simulink model "PassStCalib"  (R2024b)
settings: Solver=FixedStepDiscrete  StartTime=0.0  StopTime=10.0  FixedStep=0.01  RelTol=1e-3
model workspace (MAT data in the model file):
  KeSMSwAcsEntryPassStBkReclnUpwdDnwdPosMax_Val = Simulink.Parameter
  KeSMSwAcsEntryPassStBkReclnUpwdDnwdPosMax_Val.Value = 0
  KeSMSwAcsEntryPassStBkReclnUpwdDnwdPosMax_Val.Complexity = 'real'
  KeSMSwAcsEntryPassStBkReclnUpwdDnwdPosMax_Val.Dimensions = [1 1]
  KeSMSwAcsEntryPassStBkReclnUpwdDnwdPosMax_Val.DataType = 'uint16'
  KeSMSwAcsEntryPassStBkReclnUpwdDnwdPosMin_Val = Simulink.Parameter
  KeSMSwAcsEntryPassStBkReclnUpwdDnwdPosMin_Val.Value = 0
  KeSMSwAcsEntryPassStBkReclnUpwdDnwdPosMin_Val.Complexity = 'real'
  KeSMSwAcsEntryPassStBkReclnUpwdDnwdPosMin_Val.Dimensions = [1 1]
  KeSMSwAcsEntryPassStBkReclnUpwdDnwdPosMin_Val.DataType = 'uint16'
  KeSMSwAcsEntryPassStBkReclnUpwdDnwdPos_Val = Simulink.Parameter
  KeSMSwAcsEntryPassStBkReclnUpwdDnwdPos_Val.Value = 0
  KeSMSwAcsEntryPassStBkReclnUpwdDnwdPos_Val.Complexity = 'real'
  KeSMSwAcsEntryPassStBkReclnUpwdDnwdPos_Val.Dimensions = [1 1]
  KeSMSwAcsEntryPassStBkReclnUpwdDnwdPos_Val.DataType = 'uint16'
  KeSMSwAcsEntryPassStFrwdBkwdPosMax_Val = Simulink.Parameter
  KeSMSwAcsEntryPassStFrwdBkwdPosMax_Val.Value = 0
  KeSMSwAcsEntryPassStFrwdBkwdPosMax_Val.Complexity = 'real'
  KeSMSwAcsEntryPassStFrwdBkwdPosMax_Val.Dimensions = [1 1]
  KeSMSwAcsEntryPassStFrwdBkwdPosMax_Val.DataType = 'uint16'
  KeSMSwAcsEntryPassStFrwdBkwdPosMin_Val = Simulink.Parameter
  KeSMSwAcsEntryPassStFrwdBkwdPosMin_Val.Value = 0
  KeSMSwAcsEntryPassStFrwdBkwdPosMin_Val.Complexity = 'real'
  KeSMSwAcsEntryPassStFrwdBkwdPosMin_Val.Dimensions = [1 1]
  KeSMSwAcsEntryPassStFrwdBkwdPosMin_Val.DataType = 'uint16'
  KeSMSwAcsEntryPassStFrwdBkwdPos_Val = Simulink.Parameter
  KeSMSwAcsEntryPassStFrwdBkwdPos_Val.Value = 0
  KeSMSwAcsEntryPassStFrwdBkwdPos_Val.Complexity = 'real'
  KeSMSwAcsEntryPassStFrwdBkwdPos_Val.Dimensions = [1 1]
  KeSMSwAcsEntryPassStFrwdBkwdPos_Val.DataType = 'uint16'
  KeSMSwAcsMd56PassStBkReclnUpwdDnwdPosMax_Val = Simulink.Parameter
  KeSMSwAcsMd56PassStBkReclnUpwdDnwdPosMax_Val.Value = 0
  KeSMSwAcsMd56PassStBkReclnUpwdDnwdPosMax_Val.Complexity = 'real'
  KeSMSwAcsMd56PassStBkReclnUpwdDnwdPosMax_Val.Dimensions = [1 1]
  KeSMSwAcsMd56PassStBkReclnUpwdDnwdPosMax_Val.DataType = 'uint16'
  KeSMSwAcsMd56PassStBkReclnUpwdDnwdPosMin_Val = Simulink.Parameter
  KeSMSwAcsMd56PassStBkReclnUpwdDnwdPosMin_Val.Value = 0
  KeSMSwAcsMd56PassStBkReclnUpwdDnwdPosMin_Val.Complexity = 'real'
  KeSMSwAcsMd56PassStBkReclnUpwdDnwdPosMin_Val.Dimensions = [1 1]
  KeSMSwAcsMd56PassStBkReclnUpwdDnwdPosMin_Val.DataType = 'uint16'
  KeSMSwAcsMd56PassStBkReclnUpwdDnwdPos_Val = Simulink.Parameter
  KeSMSwAcsMd56PassStBkReclnUpwdDnwdPos_Val.Value = 0
  KeSMSwAcsMd56PassStBkReclnUpwdDnwdPos_Val.Complexity = 'real'
  KeSMSwAcsMd56PassStBkReclnUpwdDnwdPos_Val.Dimensions = [1 1]
  KeSMSwAcsMd56PassStBkReclnUpwdDnwdPos_Val.DataType = 'uint16'
  KeSMSwAcsMd56PassStFrwdBkwdPosMax_Val = Simulink.Parameter
  KeSMSwAcsMd56PassStFrwdBkwdPosMax_Val.Value = 0
  KeSMSwAcsMd56PassStFrwdBkwdPosMax_Val.Complexity = 'real'
  KeSMSwAcsMd56PassStFrwdBkwdPosMax_Val.Dimensions = [1 1]
  KeSMSwAcsMd56PassStFrwdBkwdPosMax_Val.DataType = 'uint16'
  KeSMSwAcsMd56PassStFrwdBkwdPosMin_Val = Simulink.Parameter
  KeSMSwAcsMd56PassStFrwdBkwdPosMin_Val.Value = 0
  KeSMSwAcsMd56PassStFrwdBkwdPosMin_Val.Complexity = 'real'
  KeSMSwAcsMd56PassStFrwdBkwdPosMin_Val.Dimensions = [1 1]
  KeSMSwAcsMd56PassStFrwdBkwdPosMin_Val.DataType = 'uint16'
  KeSMSwAcsMd56PassStFrwdBkwdPos_Val = Simulink.Parameter
  KeSMSwAcsMd56PassStFrwdBkwdPos_Val.Value = 0
  KeSMSwAcsMd56PassStFrwdBkwdPos_Val.Complexity = 'real'
  KeSMSwAcsMd56PassStFrwdBkwdPos_Val.Dimensions = [1 1]
  KeSMSwAcsMd56PassStFrwdBkwdPos_Val.DataType = 'uint16'
  KeSMSwRevRMDPassStBkReclnUpwdDnwdPosMax_Val = Simulink.Parameter
  KeSMSwRevRMDPassStBkReclnUpwdDnwdPosMax_Val.Value = 0
  KeSMSwRevRMDPassStBkReclnUpwdDnwdPosMax_Val.Complexity = 'real'
  KeSMSwRevRMDPassStBkReclnUpwdDnwdPosMax_Val.Dimensions = [1 1]
  KeSMSwRevRMDPassStBkReclnUpwdDnwdPosMax_Val.DataType = 'uint16'
  KeSMSwRevRMDPassStBkReclnUpwdDnwdPosMin_Val = Simulink.Parameter
  KeSMSwRevRMDPassStBkReclnUpwdDnwdPosMin_Val.Value = 0
  KeSMSwRevRMDPassStBkReclnUpwdDnwdPosMin_Val.Complexity = 'real'
  KeSMSwRevRMDPassStBkReclnUpwdDnwdPosMin_Val.Dimensions = [1 1]
  KeSMSwRevRMDPassStBkReclnUpwdDnwdPosMin_Val.DataType = 'uint16'
  KeSMSwRevRMDPassStBkReclnUpwdDnwdPos_Val = Simulink.Parameter
  KeSMSwRevRMDPassStBkReclnUpwdDnwdPos_Val.Value = 0
  KeSMSwRevRMDPassStBkReclnUpwdDnwdPos_Val.Complexity = 'real'
  KeSMSwRevRMDPassStBkReclnUpwdDnwdPos_Val.Dimensions = [1 1]
  KeSMSwRevRMDPassStBkReclnUpwdDnwdPos_Val.DataType = 'uint16'
  KeSMSwRevRMDPassStFrwdBkwdPosMax_Val = Simulink.Parameter
  KeSMSwRevRMDPassStFrwdBkwdPosMax_Val.Value = 0
  KeSMSwRevRMDPassStFrwdBkwdPosMax_Val.Complexity = 'real'
  KeSMSwRevRMDPassStFrwdBkwdPosMax_Val.Dimensions = [1 1]
  KeSMSwRevRMDPassStFrwdBkwdPosMax_Val.DataType = 'uint16'
  KeSMSwRevRMDPassStFrwdBkwdPosMin_Val = Simulink.Parameter
  KeSMSwRevRMDPassStFrwdBkwdPosMin_Val.Value = 0
  KeSMSwRevRMDPassStFrwdBkwdPosMin_Val.Complexity = 'real'
  KeSMSwRevRMDPassStFrwdBkwdPosMin_Val.Dimensions = [1 1]
  KeSMSwRevRMDPassStFrwdBkwdPosMin_Val.DataType = 'uint16'
  KeSMSwRevRMDPassStFrwdBkwdPos_Val = Simulink.Parameter
  KeSMSwRevRMDPassStFrwdBkwdPos_Val.Value = 0
  KeSMSwRevRMDPassStFrwdBkwdPos_Val.Complexity = 'real'
  KeSMSwRevRMDPassStFrwdBkwdPos_Val.Dimensions = [1 1]
  KeSMSwRevRMDPassStFrwdBkwdPos_Val.DataType = 'uint16'
undefined symbols (not defined in the file or in its folder): KeSMSuSecRwStVIPFtrstRefAngle_Val, KeSMSw6sAcsEntryPassStFtUpwdDnwdPos_Val, KeSMSw6sAcsEntryPassStFtUpwdDnwdPosMiax_Val, KeSMSw6sAcsEntryPassStFtUpwdDnwdPosMin_Val, KeSMSw6sAcsExtPassStFtUpwdDnwdPos_Val, KeSMSw6sAcsExtPassStFtUpwdDnwdPosMax_Val, KeSMSw6sAcsExtPassStFtUpwdDnwdPosMin_Val, KeSMSw6sRecoveryPassStStFtUpwdDnwdPos_Val, KeSMSw6sRecoveryPassStStFtUpwdDnwdPosMax_Val, KeSMSw6sRecoveryPassStStFtUpwdDnwdPosMin_Val, KeSMSw6SVIPMdPassStBkReclnUpwdDnwdPosPos_Val, KeSMSw6SVIPMdPassStBkReclnUpwdDnwdPosPosMax_Val, KeSMSw6SVIPMdPassStBkReclnUpwdDnwdPosPosMin_Val, KeSMSw6SVIPMdPassStFrwdBkwdPos2_Val, KeSMSw6SVIPMdPassStFrwdBkwdPosMax2_Val, KeSMSw6SVIPMdPassStFrwdBkwdPosMin2_Val, KeSMSw6SVIPMdPassStFrwdBkwdPosPos_Val, KeSMSw6SVIPMdPassStFrwdBkwdPosPosMax_Val, KeSMSw6SVIPMdPassStFrwdBkwdPosPosMin_Val, KeSMSwAcsEntryPassStFtUpwdDnwdPos_Val, KeSMSwAcsEntryPassStFtUpwdDnwdPosMiax_Val, KeSMSwAcsEntryPassStFtUpwdDnwdPosMin_Val, KeSMSwAcsExtPassStFtUpwdDnwdPos_Val, KeSMSwAcsExtPassStFtUpwdDnwdPosMax_Val, KeSMSwAcsExtPassStFtUpwdDnwdPosMin_Val, KeSMSwAcsMd30PassStBkReclnUpwdDnwdPos1_Val, KeSMSwAcsMd30PassStBkReclnUpwdDnwdPos1Max_Val, KeSMSwAcsMd30PassStBkReclnUpwdDnwdPos1Min_Val, KeSMSwAcsMd30PassStBkReclnUpwdDnwdPos_Val, KeSMSwAcsMd30PassStBkReclnUpwdDnwdPosMax_Val, KeSMSwAcsMd30PassStBkReclnUpwdDnwdPosMin_Val, KeSMSwAcsMd30PassStFldUpwdDnwdPos1_Val, KeSMSwAcsMd30PassStFldUpwdDnwdPos1Max_Val, KeSMSwAcsMd30PassStFldUpwdDnwdPos1Min_Val, KeSMSwAcsMd30PassStFldUpwdDnwdPos_Val, KeSMSwAcsMd30PassStFldUpwdDnwdPosMax_Val, KeSMSwAcsMd30PassStFldUpwdDnwdPosMin_Val, KeSMSwAcsMd30PassStFrwdBkwdPos1_Val, KeSMSwAcsMd30PassStFrwdBkwdPos1Max_Val, KeSMSwAcsMd30PassStFrwdBkwdPos1Min_Val, KeSMSwAcsMd30PassStFrwdBkwdPos_Val, KeSMSwAcsMd30PassStFrwdBkwdPosMax_Val, KeSMSwAcsMd30PassStFrwdBkwdPosMin_Val, KeSMSwAcsMd31PassStBkReclnUpwdDnwdPos1_Val, KeSMSwAcsMd31PassStBkReclnUpwdDnwdPos1Max_Val, KeSMSwAcsMd31PassStBkReclnUpwdDnwdPos1Min_Val, KeSMSwAcsMd31PassStBkReclnUpwdDnwdPos_Val, KeSMSwAcsMd31PassStBkReclnUpwdDnwdPosMax_Val, KeSMSwAcsMd31PassStBkReclnUpwdDnwdPosMin_Val, KeSMSwAcsMd31PassStFldUpwdDnwdPos_Val, KeSMSwAcsMd31PassStFldUpwdDnwdPosMax_Val, KeSMSwAcsMd31PassStFldUpwdDnwdPosMin_Val, KeSMSwAcsMd31PassStFrwdBkwdPos1_Val, KeSMSwAcsMd31PassStFrwdBkwdPos1Max_Val, KeSMSwAcsMd31PassStFrwdBkwdPos1Min_Val, KeSMSwAcsMd31PassStFrwdBkwdPos_Val, KeSMSwAcsMd31PassStFrwdBkwdPosMax_Val, KeSMSwAcsMd31PassStFrwdBkwdPosMin_Val, KeSMSwAcsMd57PassStBkReclnUpwdDnwdPosPos_Val, KeSMSwAcsMd57PassStBkReclnUpwdDnwdPosPosMax_Val ... (+34)
libraries: TrgtPosSelcLib x20
(part 1 of 3)
settings Model: ParameterArgumentNames=KeSMSwAcsEntryPassStBkReclnUpwdDnwdPosMax_Val,KeSMSwAcsEntryPassStBkReclnUpwdDnwdPosMin_Val,KeSMSwAcsEntryPassStBkReclnUpwdDnwdPos_Val,KeSMSwAcsEntryPassStFrwdBkwdPosMax_Val,KeSMSwAcsEntryPassStFrwdBkwdPosMin_Val,KeSMSwAcsEntryPassStFrwdBkwdPos_Val,KeSMSwAcsMd56PassStBkReclnUpwdDnwdPosMax_Val,KeSMSwAcsMd56PassStBkReclnUpwdDnwdPosMin_Val,KeSMSwAcsMd56PassStBkReclnUpwdDnwdPos_Val,KeSMSwAcsMd56PassStFrwdBkwdPosMax_Val,KeSMSwAcsMd56PassStFrwdBkwdPosMin_Val,KeSMSwAcsMd56PassStFrwdBkwdPos_Val,KeSMSwRevRMDPassStBkReclnUpwdDnwdPosMax_Val,KeSMSwRevRMDPassStBkReclnUpwdDnwdPosMin_Val,KeSMSwRevRMDPassStBkReclnUpwdDnwdPos_Val,KeSMSwRevRMDPassStFrwdBkwdPosMax_Val,KeSMSwRevRMDPassStFrwdBkwdPosMin_Val,KeSMSwRevRMDPassStFrwdBkwdPos_Val  Creator=sn2xws  LastModifiedBy=sn55gm
settings Model: ModifiedHistory=|
  | 2024.10.14 V3.0.0新增Md57，Md58
  | 2024.10.29 V3.0.1重新定义Unfold
  | 2024.11.6 V3.0.2 根据最新模式流程V2.6新增Md30 靠背位置1
  | 2024.11.18 V3.0.3 CR 946373 超级智享退出副驾改用Md31目标位置
  | 2024.11.27 V3.0.4 Md58 使用Md31的目标位置
  | 2024.12.11 V3.0.5 CR 953605
  | 2025.6.30 V3.13.0 新增Md61 md62
  | 25.7.31 V13.3.1 CR1100249 贵妃榻模式流程修改
settings SolverCC: AlgebraicLoopSolver=TrustRegion
settings DataIOCC: SaveFormat=StructureWithTime  ReturnWorkspaceOutputs=off
settings OptimizationCC: DefaultParameterBehavior=Inlined  EnhancedBackFolding=on  PassReuseOutputArgsAs=Individual arguments  ZeroExternalMemoryAtStartup=off  ZeroInternalMemoryAtStartup=off  OptimizeBlockOrder=speed  DifferentSizesBufferReuse=on  OptimizationCustomize=off  EfficientTunableParamExpr=on
settings DebuggingCC: ParameterTunabilityLossMsg=error  UnconnectedInputMsg=warning  UnconnectedOutputMsg=warning  UnconnectedLineMsg=warning  ArithmeticOperatorsInVariantConditions=warning
settings ModelReferenceCC: EnableRefExpFcnMdlSchedulingChecks=on
settings SFSimCC: MATLABDynamicMemAlloc=off  CustomCodeUndefinedFunction=UseInterfaceOnly
settings RTWCC: Description=AUTOSAR  SystemTargetFile=autosar.tlc  GenCodeOnly=on  TemplateMakefile=ert_default_tmf  GenerateReport=on  IncludeHyperlinkInReport=on  LaunchReport=on  DataTypeReplacement=CDataTypesFixedWidth  GenerateTraceInfo=on  GenerateTraceReport=on  GenerateTraceReportSl=on  GenerateTraceReportSf=on  GenerateTraceReportEml=on  GPUComputeCapability=3.5
settings CodeAppCC: ForceParamTrailComments=on  IgnoreCustomStorageClasses=off  OperatorAnnotations=on  SimulinkDataObjDesc=on  SFDataObjDesc=on  InsertBlockDesc=on
settings STFCustomTargetCC: TargetLangStandard=C99 (ISO)  MultiwordLength=256  ParMdlRefBuildCompliant=on  CompOptLevelCompliant=on  IncludeMdlTerminateFcn=off  CombineOutputUpdateFcns=on  SuppressErrorStatus=on  ERTCustomFileBanners=on  SupportNonFinite=off  SupportComplex=off  SupportContinuousTime=off  SupportNonInlinedSFcns=off  RemoveResetFunc=on  MATLABClassNameForMDSCustomization=Simulink.SoftwareTarget.ERTCustomization  AutosarCompliant=on  UseToolchainInfoCompliant=on  LookupTableObjectStructAxisOrder=2,1,3,4,...  LUTObjectStructOrderEvenSpacing=Size,Table,Breakpoints  SystemTargetFile=autosar.tlc
settings ERTTargetCC: TargetLangStandard=C99 (ISO)  ConcurrentExecutionCompliant=off  IncludeMdlTerminateFcn=off  SuppressErrorStatus=on  SupportNonFinite=off  SupportComplex=off  ModelStepFunctionPrototypeControlCompliant=off  CPPClassGenCompliant=off  AutosarCompliant=on  LookupTableObjectStructAxisOrder=2,1,3,4,...  LUTObjectStructOrderEvenSpacing=Size,Table,Breakpoints  ERTCustomFileTemplate=example_file_process.tlc  ERTFilePackagingFormat=Compact  BooleanTrueId=TRUE  BooleanFalseId=FALSE  DynamicArrayContainerType=coder::array

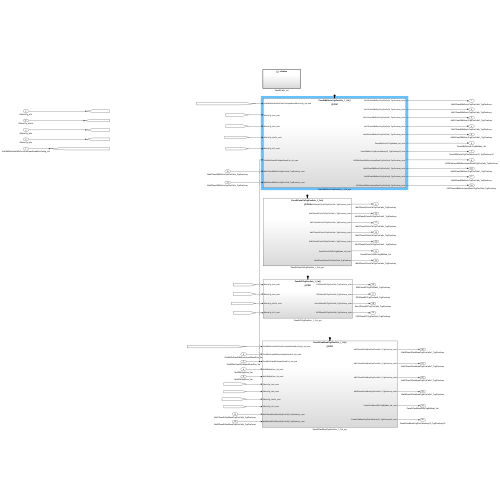
[thumbnail: Simulink's stored preview of the top-level diagram]
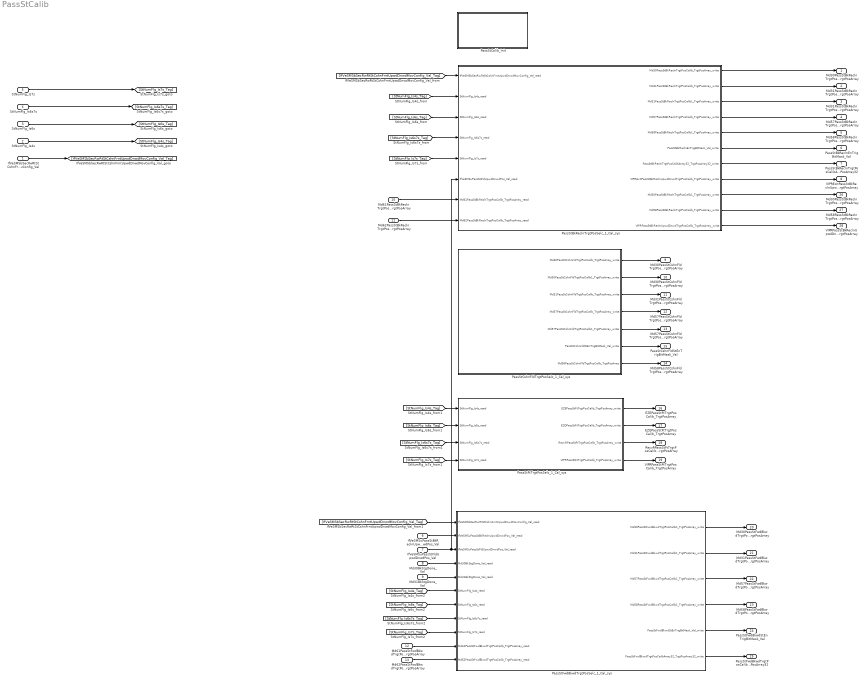
== system PassStCalib ==
  IfVeSMSbSecRwRtStCshnFrntUpwdDnwdMovConfig_Val : Inport  OutDataTypeStr=boolean  PortDimensions=1
  StNumFlg_Is4s : Inport  Port=2  OutDataTypeStr=boolean  PortDimensions=1
  StNumFlg_Is6s : Inport  Port=3  OutDataTypeStr=boolean  PortDimensions=1
  StNumFlg_Is6s7s : Inport  Port=4  OutDataTypeStr=boolean  PortDimensions=1
  StNumFlg_Is7s : Inport  Port=5  OutDataTypeStr=boolean  PortDimensions=1
  IfVeSMSuPassStBkReclnUpwdDnwdPos_Val : Inport  Port=6  OutDataTypeStr=uint16  PortDimensions=1
  IfVeSMSuPassStFldUpwdDnwdPos_Val : Inport  Port=7  OutDataTypeStr=uint16  PortDimensions=1
  Md30BkStgDone_Val : Inport  Port=8  OutDataTypeStr=boolean  PortDimensions=1
  Md31BkStgDone_Val : Inport  Port=9  OutDataTypeStr=boolean  PortDimensions=1
  Md61PassStBkReclnTrgtPosCalib_TrgtPosArray : Inport  Description=|  Port=10  OutDataTypeStr=uint16  PortDimensions=3
      | 0:Pos
      | 1:Max
      | 2:Min
  Md62PassStBkReclnTrgtPosCalib_TrgtPosArray : Inport  Description=|  Port=11  OutDataTypeStr=uint16  PortDimensions=3
      | 0:Pos
      | 1:Max
      | 2:Min
  Md61PassStFwdBkwdTrgtPosCalib_TrgtPosArray : Inport  Description=|  Port=12  OutDataTypeStr=uint16  PortDimensions=3
      | 0:Pos
      | 1:Max
      | 2:Min
  Md62PassStFwdBkwdTrgtPosCalib_TrgtPosArray : Inport  Description=|  Port=13  OutDataTypeStr=uint16  PortDimensions=3
      | 0:Pos
      | 1:Max
      | 2:Min
  PassStBkReclnTrgtPosSelc_1_Cal_sys : Subsystem
  PassStCalib_Init : Subsystem
  PassStCshnFldTrgtPosSelc_1_Cal_sys : Subsystem
  PassStFtTrgtPosSelc_1_Cal_sys : Subsystem
  PassStFwdBkwdTrgtPosSelc_1_Cal_sys : Subsystem
  Md30PassStBkReclnTrgtPosCalib_TrgtPosArray : Outport  Description=|  OutDataTypeStr=uint16  PortDimensions=3  VectorParamsAs1DForOutWhenUnconnected=off
      | 0:Pos
      | 1:Max
      | 2:Min
  Md31PassStBkReclnTrgtPosCalib_TrgtPosArray : Outport  Description=|  Port=2  OutDataTypeStr=uint16  PortDimensions=3  VectorParamsAs1DForOutWhenUnconnected=off
      | 0:Pos
      | 1:Max
      | 2:Min
  Md31PassStBkReclnTrgtPosCalib1_TrgtPosArray : Outport  Description=|  Port=3  OutDataTypeStr=uint16  PortDimensions=3  VectorParamsAs1DForOutWhenUnconnected=off
      | 0:Pos
      | 1:Max
      | 2:Min
  Md57PassStBkReclnTrgtPosCalib_TrgtPosArray : Outport  Description=|  Port=4  OutDataTypeStr=uint16  PortDimensions=3  VectorParamsAs1DForOutWhenUnconnected=off
      | 0:Pos
      | 1:Max
      | 2:Min
  Md58PassStBkReclnTrgtPosCalib1_TrgtPosArray : Outport  Description=|  Port=5  OutDataTypeStr=uint16  PortDimensions=3  VectorParamsAs1DForOutWhenUnconnected=off
      | 0:Pos
      | 1:Max
      | 2:Min
  PassStBkReclnEnTrigBitMask_Val : Outport  Port=6  OutDataTypeStr=uint32  PortDimensions=1  VectorParamsAs1DForOutWhenUnconnected=off
  PassStBkReclnTrgtPosCalibArray32_TrgtPosArray32 : Outport  Description=|  Port=7  OutDataTypeStr=uint16  PortDimensions=96  VectorParamsAs1DForOutWhenUnconnected=off
      | 0:Pos
      | 1:Max
      | 2:Min
  VIPRExitPassStBkReclnUpwdDnwdTrgtPosCalib_TrgtPosArray : Outport  Description=|  Port=8  OutDataTypeStr=uint16  PortDimensions=3  VectorParamsAs1DForOutWhenUnconnected=off
      | 0:Pos
      | 1:Max
      | 2:Min
  Md30PassStCshnFldTrgtPosCalib_TrgtPosArray : Outport  Description=|  Port=9  OutDataTypeStr=uint16  PortDimensions=3  VectorParamsAs1DForOutWhenUnconnected=off
      | 0:Pos
      | 1:Max
      | 2:Min
  Md30PassStCshnFldTrgtPosCalib1_TrgtPosArray : Outport  Description=|  Port=10  OutDataTypeStr=uint16  PortDimensions=3  VectorParamsAs1DForOutWhenUnconnected=off
      | 0:Pos
      | 1:Max
      | 2:Min
  Md31PassStCshnFldTrgtPosCalib_TrgtPosArray : Outport  Description=|  Port=11  OutDataTypeStr=uint16  PortDimensions=3  VectorParamsAs1DForOutWhenUnconnected=off
      | 0:Pos
      | 1:Max
      | 2:Min
  Md57PassStCshnFldTrgtPosCalib_TrgtPosArray : Outport  Description=|  Port=12  OutDataTypeStr=uint16  PortDimensions=3  VectorParamsAs1DForOutWhenUnconnected=off
      | 0:Pos
      | 1:Max
      | 2:Min
  Md57PassStCshnFldTrgtPosCalib1_TrgtPosArray : Outport  Description=|  Port=13  OutDataTypeStr=uint16  PortDimensions=3  VectorParamsAs1DForOutWhenUnconnected=off
      | 0:Pos
      | 1:Max
      | 2:Min
  Md58PassStCshnFldTrgtPosCalib_TrgtPosArray : Outport  Description=|  Port=14  OutDataTypeStr=uint16  PortDimensions=3  VectorParamsAs1DForOutWhenUnconnected=off
      | 0:Pos
      | 1:Max
      | 2:Min
  PassStCshnFldStEnTrigBitMask_Val : Outport  Port=15  OutDataTypeStr=uint32  PortDimensions=1  VectorParamsAs1DForOutWhenUnconnected=off
  EZEPassStFtTrgtPosCalib_TrgtPosArray : Outport  Description=|  Port=16  OutDataTypeStr=uint16  PortDimensions=3  VectorParamsAs1DForOutWhenUnconnected=off
      | 0:Pos
      | 1:Max
      | 2:Min
  EZQPassStFtTrgtPosCalib_TrgtPosArray : Outport  Description=|  Port=17  OutDataTypeStr=uint16  PortDimensions=3  VectorParamsAs1DForOutWhenUnconnected=off
      | 0:Pos
      | 1:Max
      | 2:Min
  RecvRPassStFtTrgtPosCalib_TrgtPosArray : Outport  Description=|  Port=18  OutDataTypeStr=uint16  PortDimensions=3  VectorParamsAs1DForOutWhenUnconnected=off
      | 0:Pos
      | 1:Max
      | 2:Min
  VIPRPassStFtTrgtPosCalib_TrgtPosArray : Outport  Description=|  Port=19  OutDataTypeStr=uint16  PortDimensions=3  VectorParamsAs1DForOutWhenUnconnected=off
      | 0:Pos
      | 1:Max
      | 2:Min
  Md30PassStFwdBkwdTrgtPosCalib1_TrgtPosArray : Outport  Description=|  Port=20  OutDataTypeStr=uint16  PortDimensions=3  VectorParamsAs1DForOutWhenUnconnected=off
      | 0:Pos
      | 1:Max
      | 2:Min
  Md31PassStFwdBkwdTrgtPosCalib1_TrgtPosArray : Outport  Description=|  Port=21  OutDataTypeStr=uint16  PortDimensions=3  VectorParamsAs1DForOutWhenUnconnected=off
      | 0:Pos
      | 1:Max
      | 2:Min
  Md57PassStFwdBkwdTrgtPosCalib1_TrgtPosArray : Outport  Description=|  Port=22  OutDataTypeStr=uint16  PortDimensions=3  VectorParamsAs1DForOutWhenUnconnected=off
      | 0:Pos
      | 1:Max
      | 2:Min
  Md58PassStFwdBkwdTrgtPosCalib1_TrgtPosArray : Outport  Description=|  Port=23  OutDataTypeStr=uint16  PortDimensions=3  VectorParamsAs1DForOutWhenUnconnected=off
      | 0:Pos
      | 1:Max
      | 2:Min
  PassStFwdBkwdStEnTrigBitMask_Val : Outport  Port=24  OutDataTypeStr=uint32  PortDimensions=1  VectorParamsAs1DForOutWhenUnconnected=off
  PassStFwdBkwdTrgtPosCalibArray32_TrgtPosArray32 : Outport  Description=|  Port=25  OutDataTypeStr=uint16  PortDimensions=96  VectorParamsAs1DForOutWhenUnconnected=off
      | 0:Pos
      | 1:Max
      | 2:Min
  Md30PassStBkReclnTrgtPosCalib1_TrgtPosArray : Outport  Description=|  Port=26  OutDataTypeStr=uint16  PortDimensions=3  VectorParamsAs1DForOutWhenUnconnected=off
      | 0:Pos
      | 1:Max
      | 2:Min
  Md58PassStBkReclnTrgtPosCalib_TrgtPosArray : Outport  Description=|  Port=27  OutDataTypeStr=uint16  PortDimensions=3  VectorParamsAs1DForOutWhenUnconnected=off
      | 0:Pos
      | 1:Max
      | 2:Min
  VIPRPassStBkReclnUpwdDnwdTrgtPosCalib_TrgtPosArray : Outport  Description=|  Port=28  OutDataTypeStr=uint16  PortDimensions=3  VectorParamsAs1DForOutWhenUnconnected=off
      | 0:Pos
      | 1:Max
      | 2:Min
  wires:
  PassStBkReclnTrgtPosSelc_1_Cal_sys/1(Md30PassStBkReclnTrgtPosCalib_TrgtPosArray_write) -> Md30PassStBkReclnTrgtPosCalib_TrgtPosArray/1
  PassStBkReclnTrgtPosSelc_1_Cal_sys/2(Md31PassStBkReclnTrgtPosCalib_TrgtPosArray_write) -> Md31PassStBkReclnTrgtPosCalib_TrgtPosArray/1
  PassStBkReclnTrgtPosSelc_1_Cal_sys/3(Md31PassStBkReclnTrgtPosCalib1_TrgtPosArray_write) -> Md31PassStBkReclnTrgtPosCalib1_TrgtPosArray/1
  PassStBkReclnTrgtPosSelc_1_Cal_sys/4(Md57PassStBkReclnTrgtPosCalib_TrgtPosArray_write) -> Md57PassStBkReclnTrgtPosCalib_TrgtPosArray/1
  PassStBkReclnTrgtPosSelc_1_Cal_sys/5(Md58PassStBkReclnTrgtPosCalib1_TrgtPosArray_write) -> Md58PassStBkReclnTrgtPosCalib1_TrgtPosArray/1
  PassStBkReclnTrgtPosSelc_1_Cal_sys/6(PassStBkReclnEnTrigBitMask_Val_write) -> PassStBkReclnEnTrigBitMask_Val/1
  PassStBkReclnTrgtPosSelc_1_Cal_sys/7(PassStBkReclnTrgtPosCalibArray32_TrgtPosArray32_write) -> PassStBkReclnTrgtPosCalibArray32_TrgtPosArray32/1
  PassStBkReclnTrgtPosSelc_1_Cal_sys/8(VIPRExitPassStBkReclnUpwdDnwdTrgtPosCalib_TrgtPosArray_write) -> VIPRExitPassStBkReclnUpwdDnwdTrgtPosCalib_TrgtPosArray/1
  PassStCshnFldTrgtPosSelc_1_Cal_sys/1(Md30PassStCshnFldTrgtPosCalib_TrgtPosArray_write) -> Md30PassStCshnFldTrgtPosCalib_TrgtPosArray/1
  PassStCshnFldTrgtPosSelc_1_Cal_sys/2(Md30PassStCshnFldTrgtPosCalib1_TrgtPosArray_write) -> Md30PassStCshnFldTrgtPosCalib1_TrgtPosArray/1
  PassStCshnFldTrgtPosSelc_1_Cal_sys/3(Md31PassStCshnFldTrgtPosCalib_TrgtPosArray_write) -> Md31PassStCshnFldTrgtPosCalib_TrgtPosArray/1
  PassStCshnFldTrgtPosSelc_1_Cal_sys/4(Md57PassStCshnFldTrgtPosCalib_TrgtPosArray_write) -> Md57PassStCshnFldTrgtPosCalib_TrgtPosArray/1
  PassStCshnFldTrgtPosSelc_1_Cal_sys/5(Md57PassStCshnFldTrgtPosCalib1_TrgtPosArray_write) -> Md57PassStCshnFldTrgtPosCalib1_TrgtPosArray/1
  PassStCshnFldTrgtPosSelc_1_Cal_sys/6(PassStCshnFldStEnTrigBitMask_Val_write) -> PassStCshnFldStEnTrigBitMask_Val/1
  PassStFtTrgtPosSelc_1_Cal_sys/1(EZEPassStFtTrgtPosCalib_TrgtPosArray_write) -> EZEPassStFtTrgtPosCalib_TrgtPosArray/1
  PassStFtTrgtPosSelc_1_Cal_sys/2(EZQPassStFtTrgtPosCalib_TrgtPosArray_write) -> EZQPassStFtTrgtPosCalib_TrgtPosArray/1
  PassStFtTrgtPosSelc_1_Cal_sys/3(RecvRPassStFtTrgtPosCalib_TrgtPosArray_write) -> RecvRPassStFtTrgtPosCalib_TrgtPosArray/1
  PassStFtTrgtPosSelc_1_Cal_sys/4(VIPRPassStFtTrgtPosCalib_TrgtPosArray_write) -> VIPRPassStFtTrgtPosCalib_TrgtPosArray/1
  IfVeSMSuPassStBkReclnUpwdDnwdPos_Val/1 -> PassStFwdBkwdTrgtPosSelc_1_Cal_sys/2(IfVeSMSuPassStBkReclnUpwdDnwdPos_Val_read)
  IfVeSMSuPassStFldUpwdDnwdPos_Val/1 -> PassStFwdBkwdTrgtPosSelc_1_Cal_sys/3(IfVeSMSuPassStFldUpwdDnwdPos_Val_read), PassStBkReclnTrgtPosSelc_1_Cal_sys/6(IfVeSMSuPassStFldUpwdDnwdPos_Val_read)
  Md30BkStgDone_Val/1 -> PassStFwdBkwdTrgtPosSelc_1_Cal_sys/4(Md30BkStgDone_Val_read)
  Md31BkStgDone_Val/1 -> PassStFwdBkwdTrgtPosSelc_1_Cal_sys/5(Md31BkStgDone_Val_read)
  PassStFwdBkwdTrgtPosSelc_1_Cal_sys/1(Md30PassStFwdBkwdTrgtPosCalib1_TrgtPosArray_write) -> Md30PassStFwdBkwdTrgtPosCalib1_TrgtPosArray/1
  PassStFwdBkwdTrgtPosSelc_1_Cal_sys/2(Md31PassStFwdBkwdTrgtPosCalib1_TrgtPosArray_write) -> Md31PassStFwdBkwdTrgtPosCalib1_TrgtPosArray/1
  PassStFwdBkwdTrgtPosSelc_1_Cal_sys/3(Md57PassStFwdBkwdTrgtPosCalib1_TrgtPosArray_write) -> Md57PassStFwdBkwdTrgtPosCalib1_TrgtPosArray/1
  PassStFwdBkwdTrgtPosSelc_1_Cal_sys/4(Md58PassStFwdBkwdTrgtPosCalib1_TrgtPosArray_write) -> Md58PassStFwdBkwdTrgtPosCalib1_TrgtPosArray/1
  PassStFwdBkwdTrgtPosSelc_1_Cal_sys/5(PassStFwdBkwdStEnTrigBitMask_Val_write) -> PassStFwdBkwdStEnTrigBitMask_Val/1
  PassStFwdBkwdTrgtPosSelc_1_Cal_sys/6(PassStFwdBkwdTrgtPosCalibArray32_TrgtPosArray32_write) -> PassStFwdBkwdTrgtPosCalibArray32_TrgtPosArray32/1
  StNumFlg_Is7s/1 -> [StNumFlg_Is7s_Tag]
  [StNumFlg_Is7s_Tag] -> PassStBkReclnTrgtPosSelc_1_Cal_sys/5(StNumFlg_Is7s_read)
  [StNumFlg_Is7s_Tag] -> PassStFtTrgtPosSelc_1_Cal_sys/4(StNumFlg_Is7s_read)
  [StNumFlg_Is7s_Tag] -> PassStFwdBkwdTrgtPosSelc_1_Cal_sys/9(StNumFlg_Is7s_read)
  StNumFlg_Is6s7s/1 -> [StNumFlg_Is6s7s_Tag]
  [StNumFlg_Is6s7s_Tag] -> PassStBkReclnTrgtPosSelc_1_Cal_sys/4(StNumFlg_Is6s7s_read)
  [StNumFlg_Is6s7s_Tag] -> PassStFtTrgtPosSelc_1_Cal_sys/3(StNumFlg_Is6s7s_read)
  [StNumFlg_Is6s7s_Tag] -> PassStFwdBkwdTrgtPosSelc_1_Cal_sys/8(StNumFlg_Is6s7s_read)
  StNumFlg_Is6s/1 -> [StNumFlg_Is6s_Tag]
  [StNumFlg_Is6s_Tag] -> PassStBkReclnTrgtPosSelc_1_Cal_sys/3(StNumFlg_Is6s_read)
  [StNumFlg_Is6s_Tag] -> PassStFtTrgtPosSelc_1_Cal_sys/2(StNumFlg_Is6s_read)
  [StNumFlg_Is6s_Tag] -> PassStFwdBkwdTrgtPosSelc_1_Cal_sys/7(StNumFlg_Is6s_read)
  StNumFlg_Is4s/1 -> [StNumFlg_Is4s_Tag]
  [StNumFlg_Is4s_Tag] -> PassStBkReclnTrgtPosSelc_1_Cal_sys/2(StNumFlg_Is4s_read)
  [StNumFlg_Is4s_Tag] -> PassStFtTrgtPosSelc_1_Cal_sys/1(StNumFlg_Is4s_read)
  [StNumFlg_Is4s_Tag] -> PassStFwdBkwdTrgtPosSelc_1_Cal_sys/6(StNumFlg_Is4s_read)
  IfVeSMSbSecRwRtStCshnFrntUpwdDnwdMovConfig_Val/1 -> [IfVeSMSbSecRwRtStCshnFrntUpwdDnwdMovConfig_Val_Tag]
  [IfVeSMSbSecRwRtStCshnFrntUpwdDnwdMovConfig_Val_Tag] -> PassStBkReclnTrgtPosSelc_1_Cal_sys/1(IfVeSMSbSecRwRtStCshnFrntUpwdDnwdMovConfig_Val_read)
  [IfVeSMSbSecRwRtStCshnFrntUpwdDnwdMovConfig_Val_Tag] -> PassStFwdBkwdTrgtPosSelc_1_Cal_sys/1(IfVeSMSbSecRwRtStCshnFrntUpwdDnwdMovConfig_Val_read)
  PassStBkReclnTrgtPosSelc_1_Cal_sys/9(Md30PassStBkReclnTrgtPosCalib1_TrgtPosArray_write) -> Md30PassStBkReclnTrgtPosCalib1_TrgtPosArray/1
  PassStBkReclnTrgtPosSelc_1_Cal_sys/10(Md58PassStBkReclnTrgtPosCalib_TrgtPosArray_write) -> Md58PassStBkReclnTrgtPosCalib_TrgtPosArray/1
  Md61PassStBkReclnTrgtPosCalib_TrgtPosArray/1 -> PassStBkReclnTrgtPosSelc_1_Cal_sys/7(Md61PassStBkReclnTrgtPosCalib_TrgtPosArray_read)
  Md62PassStBkReclnTrgtPosCalib_TrgtPosArray/1 -> PassStBkReclnTrgtPosSelc_1_Cal_sys/8(Md62PassStBkReclnTrgtPosCalib_TrgtPosArray_read)
  PassStBkReclnTrgtPosSelc_1_Cal_sys/11(VIPRPassStBkReclnUpwdDnwdTrgtPosCalib_TrgtPosArray_write) -> VIPRPassStBkReclnUpwdDnwdTrgtPosCalib_TrgtPosArray/1
  Md61PassStFwdBkwdTrgtPosCalib_TrgtPosArray/1 -> PassStFwdBkwdTrgtPosSelc_1_Cal_sys/10(Md61PassStFwdBkwdTrgtPosCalib_TrgtPosArray_read)
  Md62PassStFwdBkwdTrgtPosCalib_TrgtPosArray/1 -> PassStFwdBkwdTrgtPosSelc_1_Cal_sys/11(Md62PassStFwdBkwdTrgtPosCalib_TrgtPosArray_read)
  PassStCshnFldTrgtPosSelc_1_Cal_sys/7(Md58PassStCshnFldTrgtPosCalib_TrgtPosArray) -> Md58PassStCshnFldTrgtPosCalib_TrgtPosArray/1

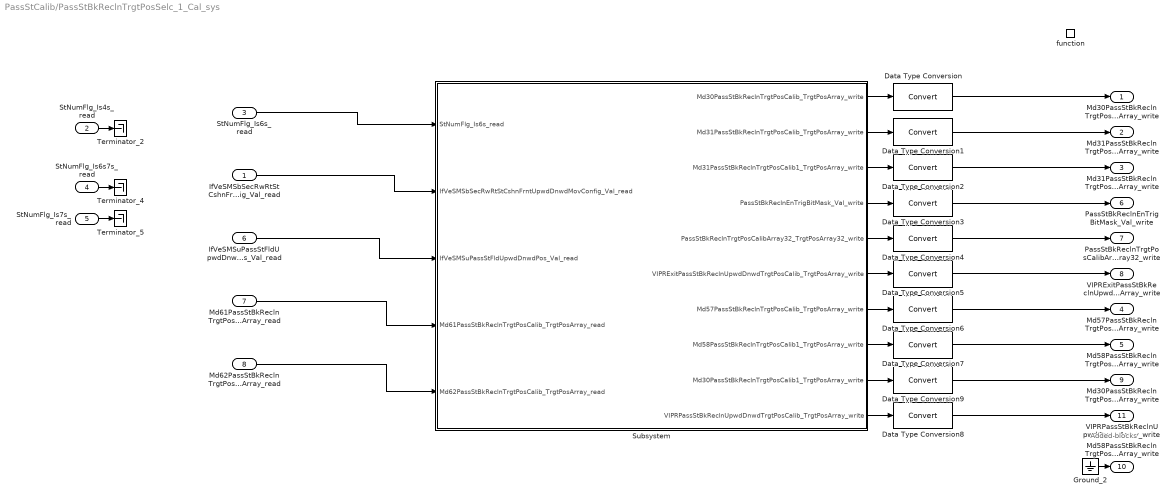
== system PassStCalib/PassStBkReclnTrgtPosSelc_1_Cal_sys ==
  note: Added blocks
  IfVeSMSbSecRwRtStCshnFrntUpwdDnwdMovConfig_Val_read : Inport
  StNumFlg_Is4s_read : Inport  Port=2
  StNumFlg_Is6s_read : Inport  Port=3
  StNumFlg_Is6s7s_read : Inport  Port=4
  StNumFlg_Is7s_read : Inport  Port=5
  IfVeSMSuPassStFldUpwdDnwdPos_Val_read : Inport  Port=6
  Md61PassStBkReclnTrgtPosCalib_TrgtPosArray_read : Inport  Port=7
  Md62PassStBkReclnTrgtPosCalib_TrgtPosArray_read : Inport  Port=8
  function : TriggerPort  TriggerType=function-call  IsSimulinkFunction=on  FunctionName=PassStBkReclnTrgtPosSelc_1_Cal  VariantControl=(inherit)
  Data Type Conversion{,1..9} (10 alike) : DataTypeConversion  SaturateOnIntegerOverflow=off  RndMeth=Floor
  Ground_2 : Ground
  Subsystem : Subsystem
  Terminator_2 : Terminator
  Terminator_4 : Terminator
  Terminator_5 : Terminator
  Md30PassStBkReclnTrgtPosCalib_TrgtPosArray_write : Outport  VectorParamsAs1DForOutWhenUnconnected=off
  Md31PassStBkReclnTrgtPosCalib_TrgtPosArray_write : Outport  Port=2  VectorParamsAs1DForOutWhenUnconnected=off
  Md31PassStBkReclnTrgtPosCalib1_TrgtPosArray_write : Outport  Port=3  VectorParamsAs1DForOutWhenUnconnected=off
  Md57PassStBkReclnTrgtPosCalib_TrgtPosArray_write : Outport  Port=4  VectorParamsAs1DForOutWhenUnconnected=off
  Md58PassStBkReclnTrgtPosCalib1_TrgtPosArray_write : Outport  Port=5  VectorParamsAs1DForOutWhenUnconnected=off
  PassStBkReclnEnTrigBitMask_Val_write : Outport  Port=6  VectorParamsAs1DForOutWhenUnconnected=off
  PassStBkReclnTrgtPosCalibArray32_TrgtPosArray32_write : Outport  Port=7  VectorParamsAs1DForOutWhenUnconnected=off
  VIPRExitPassStBkReclnUpwdDnwdTrgtPosCalib_TrgtPosArray_write : Outport  Port=8  VectorParamsAs1DForOutWhenUnconnected=off
  Md30PassStBkReclnTrgtPosCalib1_TrgtPosArray_write : Outport  Port=9  VectorParamsAs1DForOutWhenUnconnected=off
  Md58PassStBkReclnTrgtPosCalib_TrgtPosArray_write : Outport  Port=10  VectorParamsAs1DForOutWhenUnconnected=off
  VIPRPassStBkReclnUpwdDnwdTrgtPosCalib_TrgtPosArray_write : Outport  Port=11  VectorParamsAs1DForOutWhenUnconnected=off
      settings: EnsureOutportIsVirtual=on
  wires:
  IfVeSMSbSecRwRtStCshnFrntUpwdDnwdMovConfig_Val_read/1 -> Subsystem/2(IfVeSMSbSecRwRtStCshnFrntUpwdDnwdMovConfig_Val_read)
  StNumFlg_Is4s_read/1 -> Terminator_2/1
  StNumFlg_Is6s_read/1 -> Subsystem/1(StNumFlg_Is6s_read)
  StNumFlg_Is6s7s_read/1 -> Terminator_4/1
  StNumFlg_Is7s_read/1 -> Terminator_5/1
  Subsystem/1(Md30PassStBkReclnTrgtPosCalib_TrgtPosArray_write) -> Data Type Conversion/1
  Subsystem/2(Md31PassStBkReclnTrgtPosCalib_TrgtPosArray_write) -> Data Type Conversion1/1
  Subsystem/3(Md31PassStBkReclnTrgtPosCalib1_TrgtPosArray_write) -> Data Type Conversion2/1
  Subsystem/4(PassStBkReclnEnTrigBitMask_Val_write) -> Data Type Conversion3/1
  Subsystem/5(PassStBkReclnTrgtPosCalibArray32_TrgtPosArray32_write) -> Data Type Conversion4/1
  Subsystem/6(VIPRExitPassStBkReclnUpwdDnwdTrgtPosCalib_TrgtPosArray_write) -> Data Type Conversion5/1
  Subsystem/7(Md57PassStBkReclnTrgtPosCalib_TrgtPosArray_write) -> Data Type Conversion6/1
  Subsystem/8(Md58PassStBkReclnTrgtPosCalib1_TrgtPosArray_write) -> Data Type Conversion7/1
  Data Type Conversion/1 -> Md30PassStBkReclnTrgtPosCalib_TrgtPosArray_write/1
  Data Type Conversion1/1 -> Md31PassStBkReclnTrgtPosCalib_TrgtPosArray_write/1
  Data Type Conversion2/1 -> Md31PassStBkReclnTrgtPosCalib1_TrgtPosArray_write/1
  Data Type Conversion3/1 -> PassStBkReclnEnTrigBitMask_Val_write/1
  Data Type Conversion4/1 -> PassStBkReclnTrgtPosCalibArray32_TrgtPosArray32_write/1
  Data Type Conversion5/1 -> VIPRExitPassStBkReclnUpwdDnwdTrgtPosCalib_TrgtPosArray_write/1
  Data Type Conversion6/1 -> Md57PassStBkReclnTrgtPosCalib_TrgtPosArray_write/1
  Data Type Conversion7/1 -> Md58PassStBkReclnTrgtPosCalib1_TrgtPosArray_write/1
  Subsystem/9(Md30PassStBkReclnTrgtPosCalib1_TrgtPosArray_write) -> Data Type Conversion9/1
  Ground_2/1 -> Md58PassStBkReclnTrgtPosCalib_TrgtPosArray_write/1
  IfVeSMSuPassStFldUpwdDnwdPos_Val_read/1 -> Subsystem/3(IfVeSMSuPassStFldUpwdDnwdPos_Val_read)
  Data Type Conversion9/1 -> Md30PassStBkReclnTrgtPosCalib1_TrgtPosArray_write/1
  Md61PassStBkReclnTrgtPosCalib_TrgtPosArray_read/1 -> Subsystem/4(Md61PassStBkReclnTrgtPosCalib_TrgtPosArray_read)
  Md62PassStBkReclnTrgtPosCalib_TrgtPosArray_read/1 -> Subsystem/5(Md62PassStBkReclnTrgtPosCalib_TrgtPosArray_read)
  Subsystem/10(VIPRPassStBkReclnUpwdDnwdTrgtPosCalib_TrgtPosArray_write) -> Data Type Conversion8/1
  Data Type Conversion8/1 -> VIPRPassStBkReclnUpwdDnwdTrgtPosCalib_TrgtPosArray_write/1

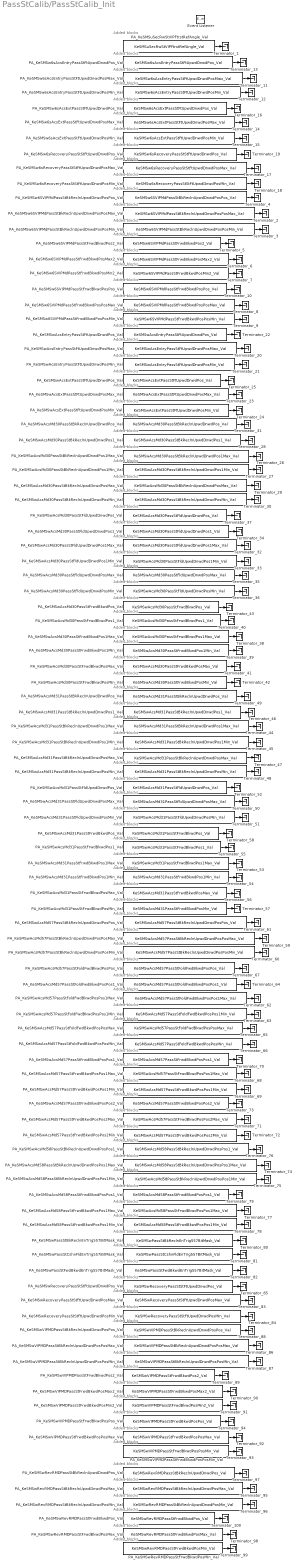
== system PassStCalib/PassStCalib_Init ==
  note: Added blocks
  note: Added blocks
  note: Added blocks
  note: Added blocks
  note: Added blocks
  note: Added blocks
  note: Added blocks
  note: Added blocks
  note: Added blocks
  note: Added blocks
  note: Added blocks
  note: Added blocks
  note: Added blocks
  note: Added blocks
  note: Added blocks
  note: Added blocks
  note: Added blocks
  note: Added blocks
  note: Added blocks
  note: Added blocks
  note: Added blocks
  note: Added blocks
  note: Added blocks
  note: Added blocks
  note: Added blocks
  note: Added blocks
  note: Added blocks
  note: Added blocks
  note: Added blocks
  note: Added blocks
  note: Added blocks
  note: Added blocks
  note: Added blocks
  note: Added blocks
  note: Added blocks
  note: Added blocks
  note: Added blocks
  note: Added blocks
  note: Added blocks
  note: Added blocks
  note: Added blocks
  note: Added blocks
  note: Added blocks
  note: Added blocks
  note: Added blocks
  note: Added blocks
  note: Added blocks
  note: Added blocks
  note: Added blocks
  note: Added blocks
  note: Added blocks
  note: Added blocks
  note: Added blocks
  note: Added blocks
  note: Added blocks
  note: Added blocks
  note: Added blocks
  note: Added blocks
  note: Added blocks
  note: Added blocks
  note: Added blocks
  note: Added blocks
  note: Added blocks
  note: Added blocks
  note: Added blocks
  note: Added blocks
  note: Added blocks
  note: Added blocks
  note: Added blocks
  note: Added blocks
  note: Added blocks
  note: Added blocks
  note: Added blocks
  note: Added blocks
  note: Added blocks
  note: Added blocks
  note: Added blocks
  note: Added blocks
  note: Added blocks
  note: Added blocks
  note: Added blocks
  note: Added blocks
  note: Added blocks
  note: Added blocks
  note: Added blocks
  note: Added blocks
  note: Added blocks
  note: Added blocks
  note: Added blocks
  note: Added blocks
  note: Added blocks
  note: Added blocks
  note: Added blocks
  note: Added blocks
  note: Added blocks
  note: Added blocks
  note: Added blocks
  note: Added blocks
  note: Added blocks
  note: Added blocks
  Event Listener : EventListener  EventName=reset
  PA_KeSMSuSecRwStVIPFtrstRefAngle_Val : Constant  Value=KeSMSuSecRwStVIPFtrstRefAngle_Val
  PA_KeSMSw6SVIPMdPassStBkReclnUpwdDnwdPosPosMax_Val : Constant  Value=KeSMSw6SVIPMdPassStBkReclnUpwdDnwdPosPosMax_Val
  PA_KeSMSw6SVIPMdPassStBkReclnUpwdDnwdPosPosMin_Val : Constant  Value=KeSMSw6SVIPMdPassStBkReclnUpwdDnwdPosPosMin_Val
  PA_KeSMSw6SVIPMdPassStBkReclnUpwdDnwdPosPos_Val : Constant  Value=KeSMSw6SVIPMdPassStBkReclnUpwdDnwdPosPos_Val
  PA_KeSMSw6SVIPMdPassStFrwdBkwdPos2_Val : Constant  Value=KeSMSw6SVIPMdPassStFrwdBkwdPos2_Val
  PA_KeSMSw6SVIPMdPassStFrwdBkwdPosMax2_Val : Constant  Value=KeSMSw6SVIPMdPassStFrwdBkwdPosMax2_Val
  PA_KeSMSw6SVIPMdPassStFrwdBkwdPosMin2_Val : Constant  Value=KeSMSw6SVIPMdPassStFrwdBkwdPosMin2_Val
  PA_KeSMSw6SVIPMdPassStFrwdBkwdPosPosMax_Val : Constant  Value=KeSMSw6SVIPMdPassStFrwdBkwdPosPosMax_Val
  PA_KeSMSw6SVIPMdPassStFrwdBkwdPosPosMin_Val : Constant  Value=KeSMSw6SVIPMdPassStFrwdBkwdPosPosMin_Val
  PA_KeSMSw6SVIPMdPassStFrwdBkwdPosPos_Val : Constant  Value=KeSMSw6SVIPMdPassStFrwdBkwdPosPos_Val
  PA_KeSMSw6sAcsEntryPassStFtUpwdDnwdPosMiax_Val : Constant  Value=KeSMSw6sAcsEntryPassStFtUpwdDnwdPosMiax_Val
  PA_KeSMSw6sAcsEntryPassStFtUpwdDnwdPosMin_Val : Constant  Value=KeSMSw6sAcsEntryPassStFtUpwdDnwdPosMin_Val
  PA_KeSMSw6sAcsEntryPassStFtUpwdDnwdPos_Val : Constant  Value=KeSMSw6sAcsEntryPassStFtUpwdDnwdPos_Val
  PA_KeSMSw6sAcsExtPassStFtUpwdDnwdPosMax_Val : Constant  Value=KeSMSw6sAcsExtPassStFtUpwdDnwdPosMax_Val
  PA_KeSMSw6sAcsExtPassStFtUpwdDnwdPosMin_Val : Constant  Value=KeSMSw6sAcsExtPassStFtUpwdDnwdPosMin_Val
  PA_KeSMSw6sAcsExtPassStFtUpwdDnwdPos_Val : Constant  Value=KeSMSw6sAcsExtPassStFtUpwdDnwdPos_Val
  PA_KeSMSw6sRecoveryPassStStFtUpwdDnwdPosMax_Val : Constant  Value=KeSMSw6sRecoveryPassStStFtUpwdDnwdPosMax_Val
  PA_KeSMSw6sRecoveryPassStStFtUpwdDnwdPosMin_Val : Constant  Value=KeSMSw6sRecoveryPassStStFtUpwdDnwdPosMin_Val
  PA_KeSMSw6sRecoveryPassStStFtUpwdDnwdPos_Val : Constant  Value=KeSMSw6sRecoveryPassStStFtUpwdDnwdPos_Val
  PA_KeSMSwAcsEntryPassStFtUpwdDnwdPosMiax_Val : Constant  Value=KeSMSwAcsEntryPassStFtUpwdDnwdPosMiax_Val
  PA_KeSMSwAcsEntryPassStFtUpwdDnwdPosMin_Val : Constant  Value=KeSMSwAcsEntryPassStFtUpwdDnwdPosMin_Val
  PA_KeSMSwAcsEntryPassStFtUpwdDnwdPos_Val : Constant  Value=KeSMSwAcsEntryPassStFtUpwdDnwdPos_Val
  PA_KeSMSwAcsExtPassStFtUpwdDnwdPosMax_Val : Constant  Value=KeSMSwAcsExtPassStFtUpwdDnwdPosMax_Val
  PA_KeSMSwAcsExtPassStFtUpwdDnwdPosMin_Val : Constant  Value=KeSMSwAcsExtPassStFtUpwdDnwdPosMin_Val
  PA_KeSMSwAcsExtPassStFtUpwdDnwdPos_Val : Constant  Value=KeSMSwAcsExtPassStFtUpwdDnwdPos_Val
  PA_KeSMSwAcsMd30PassStBkReclnUpwdDnwdPos1Max_Val : Constant  Value=KeSMSwAcsMd30PassStBkReclnUpwdDnwdPos1Max_Val
  PA_KeSMSwAcsMd30PassStBkReclnUpwdDnwdPos1Min_Val : Constant  Value=KeSMSwAcsMd30PassStBkReclnUpwdDnwdPos1Min_Val
  PA_KeSMSwAcsMd30PassStBkReclnUpwdDnwdPos1_Val : Constant  Value=KeSMSwAcsMd30PassStBkReclnUpwdDnwdPos1_Val
  PA_KeSMSwAcsMd30PassStBkReclnUpwdDnwdPosMax_Val : Constant  Value=KeSMSwAcsMd30PassStBkReclnUpwdDnwdPosMax_Val
  PA_KeSMSwAcsMd30PassStBkReclnUpwdDnwdPosMin_Val : Constant  Value=KeSMSwAcsMd30PassStBkReclnUpwdDnwdPosMin_Val
  PA_KeSMSwAcsMd30PassStBkReclnUpwdDnwdPos_Val : Constant  Value=KeSMSwAcsMd30PassStBkReclnUpwdDnwdPos_Val
  PA_KeSMSwAcsMd30PassStFldUpwdDnwdPos1Max_Val : Constant  Value=KeSMSwAcsMd30PassStFldUpwdDnwdPos1Max_Val
  PA_KeSMSwAcsMd30PassStFldUpwdDnwdPos1Min_Val : Constant  Value=KeSMSwAcsMd30PassStFldUpwdDnwdPos1Min_Val
  PA_KeSMSwAcsMd30PassStFldUpwdDnwdPos1_Val : Constant  Value=KeSMSwAcsMd30PassStFldUpwdDnwdPos1_Val
  PA_KeSMSwAcsMd30PassStFldUpwdDnwdPosMax_Val : Constant  Value=KeSMSwAcsMd30PassStFldUpwdDnwdPosMax_Val
  PA_KeSMSwAcsMd30PassStFldUpwdDnwdPosMin_Val : Constant  Value=KeSMSwAcsMd30PassStFldUpwdDnwdPosMin_Val
  PA_KeSMSwAcsMd30PassStFldUpwdDnwdPos_Val : Constant  Value=KeSMSwAcsMd30PassStFldUpwdDnwdPos_Val
  PA_KeSMSwAcsMd30PassStFrwdBkwdPos1Max_Val : Constant  Value=KeSMSwAcsMd30PassStFrwdBkwdPos1Max_Val
  PA_KeSMSwAcsMd30PassStFrwdBkwdPos1Min_Val : Constant  Value=KeSMSwAcsMd30PassStFrwdBkwdPos1Min_Val
  PA_KeSMSwAcsMd30PassStFrwdBkwdPos1_Val : Constant  Value=KeSMSwAcsMd30PassStFrwdBkwdPos1_Val
  PA_KeSMSwAcsMd30PassStFrwdBkwdPosMax_Val : Constant  Value=KeSMSwAcsMd30PassStFrwdBkwdPosMax_Val
  PA_KeSMSwAcsMd30PassStFrwdBkwdPosMin_Val : Constant  Value=KeSMSwAcsMd30PassStFrwdBkwdPosMin_Val
  PA_KeSMSwAcsMd30PassStFrwdBkwdPos_Val : Constant  Value=KeSMSwAcsMd30PassStFrwdBkwdPos_Val
  PA_KeSMSwAcsMd31PassStBkReclnUpwdDnwdPos1Max_Val : Constant  Value=KeSMSwAcsMd31PassStBkReclnUpwdDnwdPos1Max_Val
  PA_KeSMSwAcsMd31PassStBkReclnUpwdDnwdPos1Min_Val : Constant  Value=KeSMSwAcsMd31PassStBkReclnUpwdDnwdPos1Min_Val
  PA_KeSMSwAcsMd31PassStBkReclnUpwdDnwdPos1_Val : Constant  Value=KeSMSwAcsMd31PassStBkReclnUpwdDnwdPos1_Val
  PA_KeSMSwAcsMd31PassStBkReclnUpwdDnwdPosMax_Val : Constant  Value=KeSMSwAcsMd31PassStBkReclnUpwdDnwdPosMax_Val
  PA_KeSMSwAcsMd31PassStBkReclnUpwdDnwdPosMin_Val : Constant  Value=KeSMSwAcsMd31PassStBkReclnUpwdDnwdPosMin_Val
  PA_KeSMSwAcsMd31PassStBkReclnUpwdDnwdPos_Val : Constant  Value=KeSMSwAcsMd31PassStBkReclnUpwdDnwdPos_Val
  PA_KeSMSwAcsMd31PassStFldUpwdDnwdPosMax_Val : Constant  Value=KeSMSwAcsMd31PassStFldUpwdDnwdPosMax_Val
  PA_KeSMSwAcsMd31PassStFldUpwdDnwdPosMin_Val : Constant  Value=KeSMSwAcsMd31PassStFldUpwdDnwdPosMin_Val
  PA_KeSMSwAcsMd31PassStFldUpwdDnwdPos_Val : Constant  Value=KeSMSwAcsMd31PassStFldUpwdDnwdPos_Val
  PA_KeSMSwAcsMd31PassStFrwdBkwdPos1Max_Val : Constant  Value=KeSMSwAcsMd31PassStFrwdBkwdPos1Max_Val
  PA_KeSMSwAcsMd31PassStFrwdBkwdPos1Min_Val : Constant  Value=KeSMSwAcsMd31PassStFrwdBkwdPos1Min_Val
  PA_KeSMSwAcsMd31PassStFrwdBkwdPos1_Val : Constant  Value=KeSMSwAcsMd31PassStFrwdBkwdPos1_Val
  PA_KeSMSwAcsMd31PassStFrwdBkwdPosMax_Val : Constant  Value=KeSMSwAcsMd31PassStFrwdBkwdPosMax_Val
  PA_KeSMSwAcsMd31PassStFrwdBkwdPosMin_Val : Constant  Value=KeSMSwAcsMd31PassStFrwdBkwdPosMin_Val
  PA_KeSMSwAcsMd31PassStFrwdBkwdPos_Val : Constant  Value=KeSMSwAcsMd31PassStFrwdBkwdPos_Val
  PA_KeSMSwAcsMd57PassStBkReclnUpwdDnwdPosPosMax_Val : Constant  Value=KeSMSwAcsMd57PassStBkReclnUpwdDnwdPosPosMax_Val
  PA_KeSMSwAcsMd57PassStBkReclnUpwdDnwdPosPosMin_Val : Constant  Value=KeSMSwAcsMd57PassStBkReclnUpwdDnwdPosPosMin_Val
  PA_KeSMSwAcsMd57PassStBkReclnUpwdDnwdPosPos_Val : Constant  Value=KeSMSwAcsMd57PassStBkReclnUpwdDnwdPosPos_Val
  PA_KeSMSwAcsMd57PassStFoldFwdBkwdPosPos1Max_Val : Constant  Value=KeSMSwAcsMd57PassStFoldFwdBkwdPosPos1Max_Val
  PA_KeSMSwAcsMd57PassStFoldFwdBkwdPosPos1Min_Val : Constant  Value=KeSMSwAcsMd57PassStFoldFwdBkwdPosPos1Min_Val
  PA_KeSMSwAcsMd57PassStFoldFwdBkwdPosPos1_Val : Constant  Value=KeSMSwAcsMd57PassStFoldFwdBkwdPosPos1_Val
  PA_KeSMSwAcsMd57PassStFoldFwdBkwdPosPosMax_Val : Constant  Value=KeSMSwAcsMd57PassStFoldFwdBkwdPosPosMax_Val
  PA_KeSMSwAcsMd57PassStFoldFwdBkwdPosPosMin_Val : Constant  Value=KeSMSwAcsMd57PassStFoldFwdBkwdPosPosMin_Val
  PA_KeSMSwAcsMd57PassStFoldFwdBkwdPosPos_Val : Constant  Value=KeSMSwAcsMd57PassStFoldFwdBkwdPosPos_Val
  PA_KeSMSwAcsMd57PassStFrwdBkwdPosPos1Max_Val : Constant  Value=KeSMSwAcsMd57PassStFrwdBkwdPosPos1Max_Val
  PA_KeSMSwAcsMd57PassStFrwdBkwdPosPos1Min_Val : Constant  Value=KeSMSwAcsMd57PassStFrwdBkwdPosPos1Min_Val
  PA_KeSMSwAcsMd57PassStFrwdBkwdPosPos1_Val : Constant  Value=KeSMSwAcsMd57PassStFrwdBkwdPosPos1_Val
  PA_KeSMSwAcsMd57PassStFrwdBkwdPosPos2Max_Val : Constant  Value=KeSMSwAcsMd57PassStFrwdBkwdPosPos2Max_Val
  PA_KeSMSwAcsMd57PassStFrwdBkwdPosPos2Min_Val : Constant  Value=KeSMSwAcsMd57PassStFrwdBkwdPosPos2Min_Val
  PA_KeSMSwAcsMd57PassStFrwdBkwdPosPos2_Val : Constant  Value=KeSMSwAcsMd57PassStFrwdBkwdPosPos2_Val
  PA_KeSMSwAcsMd58PassStBkReclnUpwdDnwdPosPos1Max_Val : Constant  Value=KeSMSwAcsMd58PassStBkReclnUpwdDnwdPosPos1Max_Val
  PA_KeSMSwAcsMd58PassStBkReclnUpwdDnwdPosPos1Min_Val : Constant  Value=KeSMSwAcsMd58PassStBkReclnUpwdDnwdPosPos1Min_Val
  PA_KeSMSwAcsMd58PassStBkReclnUpwdDnwdPosPos1_Val : Constant  Value=KeSMSwAcsMd58PassStBkReclnUpwdDnwdPosPos1_Val
  PA_KeSMSwAcsMd58PassStFrwdBkwdPosPos1Max_Val : Constant  Value=KeSMSwAcsMd58PassStFrwdBkwdPosPos1Max_Val
  PA_KeSMSwAcsMd58PassStFrwdBkwdPosPos1Min_Val : Constant  Value=KeSMSwAcsMd58PassStFrwdBkwdPosPos1Min_Val
  PA_KeSMSwAcsMd58PassStFrwdBkwdPosPos1_Val : Constant  Value=KeSMSwAcsMd58PassStFrwdBkwdPosPos1_Val
  PA_KeSMSwPassStBkReclnEnTrig557BitMask_Val : Constant  Value=KeSMSwPassStBkReclnEnTrig557BitMask_Val
  PA_KeSMSwPassStCshnFldEnTrig557BitMask_Val : Constant  Value=KeSMSwPassStCshnFldEnTrig557BitMask_Val
  PA_KeSMSwPassStFwdBkwdEnTrig557BitMask_Val : Constant  Value=KeSMSwPassStFwdBkwdEnTrig557BitMask_Val
  PA_KeSMSwRecoveryPassStStFtUpwdDnwdPosMax_Val : Constant  Value=KeSMSwRecoveryPassStStFtUpwdDnwdPosMax_Val
  PA_KeSMSwRecoveryPassStStFtUpwdDnwdPosMin_Val : Constant  Value=KeSMSwRecoveryPassStStFtUpwdDnwdPosMin_Val
  PA_KeSMSwRecoveryPassStStFtUpwdDnwdPos_Val : Constant  Value=KeSMSwRecoveryPassStStFtUpwdDnwdPos_Val
  PA_KeSMSwRevRMDPassStBkReclnUpwdDnwdPosMax_Val : Constant  Value=KeSMSwRevRMDPassStBkReclnUpwdDnwdPosMax_Val
  PA_KeSMSwRevRMDPassStBkReclnUpwdDnwdPosMin_Val : Constant  Value=KeSMSwRevRMDPassStBkReclnUpwdDnwdPosMin_Val
  PA_KeSMSwRevRMDPassStBkReclnUpwdDnwdPos_Val : Constant  Value=KeSMSwRevRMDPassStBkReclnUpwdDnwdPos_Val
  PA_KeSMSwRevRMDPassStFrwdBkwdPosMax_Val : Constant  Value=KeSMSwRevRMDPassStFrwdBkwdPosMax_Val
  PA_KeSMSwRevRMDPassStFrwdBkwdPosMin_Val : Constant  Value=KeSMSwRevRMDPassStFrwdBkwdPosMin_Val
  PA_KeSMSwRevRMDPassStFrwdBkwdPos_Val : Constant  Value=KeSMSwRevRMDPassStFrwdBkwdPos_Val
  PA_KeSMSwVIPMDPassStBkReclnUpwdDnwdPosPosMax_Val : Constant  Value=KeSMSwVIPMDPassStBkReclnUpwdDnwdPosPosMax_Val
  PA_KeSMSwVIPMDPassStBkReclnUpwdDnwdPosPosMin_Val : Constant  Value=KeSMSwVIPMDPassStBkReclnUpwdDnwdPosPosMin_Val
  PA_KeSMSwVIPMDPassStBkReclnUpwdDnwdPosPos_Val : Constant  Value=KeSMSwVIPMDPassStBkReclnUpwdDnwdPosPos_Val
  PA_KeSMSwVIPMDPassStFrwdBkwdPos2_Val : Constant  Value=KeSMSwVIPMDPassStFrwdBkwdPos2_Val
  PA_KeSMSwVIPMDPassStFrwdBkwdPosMax2_Val : Constant  Value=KeSMSwVIPMDPassStFrwdBkwdPosMax2_Val
  PA_KeSMSwVIPMDPassStFrwdBkwdPosMin2_Val : Constant  Value=KeSMSwVIPMDPassStFrwdBkwdPosMin2_Val
  PA_KeSMSwVIPMDPassStFrwdBkwdPosPosMax_Val : Constant  Value=KeSMSwVIPMDPassStFrwdBkwdPosPosMax_Val
  PA_KeSMSwVIPMDPassStFrwdBkwdPosPosMin_Val : Constant  Value=KeSMSwVIPMDPassStFrwdBkwdPosPosMin_Val
  PA_KeSMSwVIPMDPassStFrwdBkwdPosPos_Val : Constant  Value=KeSMSwVIPMDPassStFrwdBkwdPosPos_Val
  Terminator_{1..100} (100 alike) : Terminator
  wires:
  PA_KeSMSuSecRwStVIPFtrstRefAngle_Val/1 -> Terminator_1/1
  PA_KeSMSw6SVIPMdPassStBkReclnUpwdDnwdPosPosMax_Val/1 -> Terminator_2/1
  PA_KeSMSw6SVIPMdPassStBkReclnUpwdDnwdPosPosMin_Val/1 -> Terminator_3/1
  PA_KeSMSw6SVIPMdPassStBkReclnUpwdDnwdPosPos_Val/1 -> Terminator_4/1
  PA_KeSMSw6SVIPMdPassStFrwdBkwdPos2_Val/1 -> Terminator_5/1
  PA_KeSMSw6SVIPMdPassStFrwdBkwdPosMax2_Val/1 -> Terminator_6/1
  PA_KeSMSw6SVIPMdPassStFrwdBkwdPosMin2_Val/1 -> Terminator_7/1
  PA_KeSMSw6SVIPMdPassStFrwdBkwdPosPosMax_Val/1 -> Terminator_8/1
  PA_KeSMSw6SVIPMdPassStFrwdBkwdPosPosMin_Val/1 -> Terminator_9/1
  PA_KeSMSw6SVIPMdPassStFrwdBkwdPosPos_Val/1 -> Terminator_10/1
  PA_KeSMSw6sAcsEntryPassStFtUpwdDnwdPosMiax_Val/1 -> Terminator_11/1
  PA_KeSMSw6sAcsEntryPassStFtUpwdDnwdPosMin_Val/1 -> Terminator_12/1
  PA_KeSMSw6sAcsEntryPassStFtUpwdDnwdPos_Val/1 -> Terminator_13/1
  PA_KeSMSw6sAcsExtPassStFtUpwdDnwdPosMax_Val/1 -> Terminator_14/1
  PA_KeSMSw6sAcsExtPassStFtUpwdDnwdPosMin_Val/1 -> Terminator_15/1
  PA_KeSMSw6sAcsExtPassStFtUpwdDnwdPos_Val/1 -> Terminator_16/1
  PA_KeSMSw6sRecoveryPassStStFtUpwdDnwdPosMax_Val/1 -> Terminator_17/1
  PA_KeSMSw6sRecoveryPassStStFtUpwdDnwdPosMin_Val/1 -> Terminator_18/1
  PA_KeSMSw6sRecoveryPassStStFtUpwdDnwdPos_Val/1 -> Terminator_19/1
  PA_KeSMSwAcsEntryPassStFtUpwdDnwdPosMiax_Val/1 -> Terminator_20/1
  PA_KeSMSwAcsEntryPassStFtUpwdDnwdPosMin_Val/1 -> Terminator_21/1
  PA_KeSMSwAcsEntryPassStFtUpwdDnwdPos_Val/1 -> Terminator_22/1
  PA_KeSMSwAcsExtPassStFtUpwdDnwdPosMax_Val/1 -> Terminator_23/1
  PA_KeSMSwAcsExtPassStFtUpwdDnwdPosMin_Val/1 -> Terminator_24/1
  PA_KeSMSwAcsExtPassStFtUpwdDnwdPos_Val/1 -> Terminator_25/1
  PA_KeSMSwAcsMd30PassStBkReclnUpwdDnwdPos1Max_Val/1 -> Terminator_26/1
  PA_KeSMSwAcsMd30PassStBkReclnUpwdDnwdPos1Min_Val/1 -> Terminator_27/1
  PA_KeSMSwAcsMd30PassStBkReclnUpwdDnwdPos1_Val/1 -> Terminator_28/1
  PA_KeSMSwAcsMd30PassStBkReclnUpwdDnwdPosMax_Val/1 -> Terminator_29/1
  PA_KeSMSwAcsMd30PassStBkReclnUpwdDnwdPosMin_Val/1 -> Terminator_30/1
  PA_KeSMSwAcsMd30PassStBkReclnUpwdDnwdPos_Val/1 -> Terminator_31/1
  PA_KeSMSwAcsMd30PassStFldUpwdDnwdPos1Max_Val/1 -> Terminator_32/1
  PA_KeSMSwAcsMd30PassStFldUpwdDnwdPos1Min_Val/1 -> Terminator_33/1
  PA_KeSMSwAcsMd30PassStFldUpwdDnwdPos1_Val/1 -> Terminator_34/1
  PA_KeSMSwAcsMd30PassStFldUpwdDnwdPosMax_Val/1 -> Terminator_35/1
  PA_KeSMSwAcsMd30PassStFldUpwdDnwdPosMin_Val/1 -> Terminator_36/1
  PA_KeSMSwAcsMd30PassStFldUpwdDnwdPos_Val/1 -> Terminator_37/1
  PA_KeSMSwAcsMd30PassStFrwdBkwdPos1Max_Val/1 -> Terminator_38/1
  PA_KeSMSwAcsMd30PassStFrwdBkwdPos1Min_Val/1 -> Terminator_39/1
  PA_KeSMSwAcsMd30PassStFrwdBkwdPos1_Val/1 -> Terminator_40/1
  PA_KeSMSwAcsMd30PassStFrwdBkwdPosMax_Val/1 -> Terminator_41/1
  PA_KeSMSwAcsMd30PassStFrwdBkwdPosMin_Val/1 -> Terminator_42/1
  PA_KeSMSwAcsMd30PassStFrwdBkwdPos_Val/1 -> Terminator_43/1
  PA_KeSMSwAcsMd31PassStBkReclnUpwdDnwdPos1Max_Val/1 -> Terminator_44/1
  PA_KeSMSwAcsMd31PassStBkReclnUpwdDnwdPos1Min_Val/1 -> Terminator_45/1
  PA_KeSMSwAcsMd31PassStBkReclnUpwdDnwdPos1_Val/1 -> Terminator_46/1
  PA_KeSMSwAcsMd31PassStBkReclnUpwdDnwdPosMax_Val/1 -> Terminator_47/1
  PA_KeSMSwAcsMd31PassStBkReclnUpwdDnwdPosMin_Val/1 -> Terminator_48/1
  PA_KeSMSwAcsMd31PassStBkReclnUpwdDnwdPos_Val/1 -> Terminator_49/1
  PA_KeSMSwAcsMd31PassStFldUpwdDnwdPosMax_Val/1 -> Terminator_50/1
  PA_KeSMSwAcsMd31PassStFldUpwdDnwdPosMin_Val/1 -> Terminator_51/1
  PA_KeSMSwAcsMd31PassStFldUpwdDnwdPos_Val/1 -> Terminator_52/1
  PA_KeSMSwAcsMd31PassStFrwdBkwdPos1Max_Val/1 -> Terminator_53/1
  PA_KeSMSwAcsMd31PassStFrwdBkwdPos1Min_Val/1 -> Terminator_54/1
  PA_KeSMSwAcsMd31PassStFrwdBkwdPos1_Val/1 -> Terminator_55/1
  PA_KeSMSwAcsMd31PassStFrwdBkwdPosMax_Val/1 -> Terminator_56/1
  PA_KeSMSwAcsMd31PassStFrwdBkwdPosMin_Val/1 -> Terminator_57/1
  PA_KeSMSwAcsMd31PassStFrwdBkwdPos_Val/1 -> Terminator_58/1
  PA_KeSMSwAcsMd57PassStBkReclnUpwdDnwdPosPosMax_Val/1 -> Terminator_59/1
  PA_KeSMSwAcsMd57PassStBkReclnUpwdDnwdPosPosMin_Val/1 -> Terminator_60/1
  PA_KeSMSwAcsMd57PassStBkReclnUpwdDnwdPosPos_Val/1 -> Terminator_61/1
  PA_KeSMSwAcsMd57PassStFoldFwdBkwdPosPos1Max_Val/1 -> Terminator_62/1
  PA_KeSMSwAcsMd57PassStFoldFwdBkwdPosPos1Min_Val/1 -> Terminator_63/1
  PA_KeSMSwAcsMd57PassStFoldFwdBkwdPosPos1_Val/1 -> Terminator_64/1
  PA_KeSMSwAcsMd57PassStFoldFwdBkwdPosPosMax_Val/1 -> Terminator_65/1
  PA_KeSMSwAcsMd57PassStFoldFwdBkwdPosPosMin_Val/1 -> Terminator_66/1
  PA_KeSMSwAcsMd57PassStFoldFwdBkwdPosPos_Val/1 -> Terminator_67/1
  PA_KeSMSwAcsMd57PassStFrwdBkwdPosPos1Max_Val/1 -> Terminator_68/1
  PA_KeSMSwAcsMd57PassStFrwdBkwdPosPos1Min_Val/1 -> Terminator_69/1
  PA_KeSMSwAcsMd57PassStFrwdBkwdPosPos1_Val/1 -> Terminator_70/1
  PA_KeSMSwAcsMd57PassStFrwdBkwdPosPos2Max_Val/1 -> Terminator_71/1
  PA_KeSMSwAcsMd57PassStFrwdBkwdPosPos2Min_Val/1 -> Terminator_72/1
  PA_KeSMSwAcsMd57PassStFrwdBkwdPosPos2_Val/1 -> Terminator_73/1
  PA_KeSMSwAcsMd58PassStBkReclnUpwdDnwdPosPos1Max_Val/1 -> Terminator_74/1
  PA_KeSMSwAcsMd58PassStBkReclnUpwdDnwdPosPos1Min_Val/1 -> Terminator_75/1
  PA_KeSMSwAcsMd58PassStBkReclnUpwdDnwdPosPos1_Val/1 -> Terminator_76/1
  PA_KeSMSwAcsMd58PassStFrwdBkwdPosPos1Max_Val/1 -> Terminator_77/1
  PA_KeSMSwAcsMd58PassStFrwdBkwdPosPos1Min_Val/1 -> Terminator_78/1
  PA_KeSMSwAcsMd58PassStFrwdBkwdPosPos1_Val/1 -> Terminator_79/1
  PA_KeSMSwPassStBkReclnEnTrig557BitMask_Val/1 -> Terminator_80/1
  PA_KeSMSwPassStCshnFldEnTrig557BitMask_Val/1 -> Terminator_81/1
  PA_KeSMSwPassStFwdBkwdEnTrig557BitMask_Val/1 -> Terminator_82/1
  PA_KeSMSwRecoveryPassStStFtUpwdDnwdPosMax_Val/1 -> Terminator_83/1
  PA_KeSMSwRecoveryPassStStFtUpwdDnwdPosMin_Val/1 -> Terminator_84/1
  PA_KeSMSwRecoveryPassStStFtUpwdDnwdPos_Val/1 -> Terminator_85/1
  PA_KeSMSwVIPMDPassStBkReclnUpwdDnwdPosPosMax_Val/1 -> Terminator_86/1
  PA_KeSMSwVIPMDPassStBkReclnUpwdDnwdPosPosMin_Val/1 -> Terminator_87/1
  PA_KeSMSwVIPMDPassStBkReclnUpwdDnwdPosPos_Val/1 -> Terminator_88/1
  PA_KeSMSwVIPMDPassStFrwdBkwdPos2_Val/1 -> Terminator_89/1
  PA_KeSMSwVIPMDPassStFrwdBkwdPosMax2_Val/1 -> Terminator_90/1
  PA_KeSMSwVIPMDPassStFrwdBkwdPosMin2_Val/1 -> Terminator_91/1
  PA_KeSMSwVIPMDPassStFrwdBkwdPosPosMax_Val/1 -> Terminator_92/1
  PA_KeSMSwVIPMDPassStFrwdBkwdPosPosMin_Val/1 -> Terminator_93/1
  PA_KeSMSwVIPMDPassStFrwdBkwdPosPos_Val/1 -> Terminator_94/1
  PA_KeSMSwRevRMDPassStBkReclnUpwdDnwdPosMax_Val/1 -> Terminator_95/1
  PA_KeSMSwRevRMDPassStBkReclnUpwdDnwdPosMin_Val/1 -> Terminator_96/1
  PA_KeSMSwRevRMDPassStBkReclnUpwdDnwdPos_Val/1 -> Terminator_97/1
  PA_KeSMSwRevRMDPassStFrwdBkwdPosMax_Val/1 -> Terminator_98/1
  PA_KeSMSwRevRMDPassStFrwdBkwdPosMin_Val/1 -> Terminator_99/1
  PA_KeSMSwRevRMDPassStFrwdBkwdPos_Val/1 -> Terminator_100/1

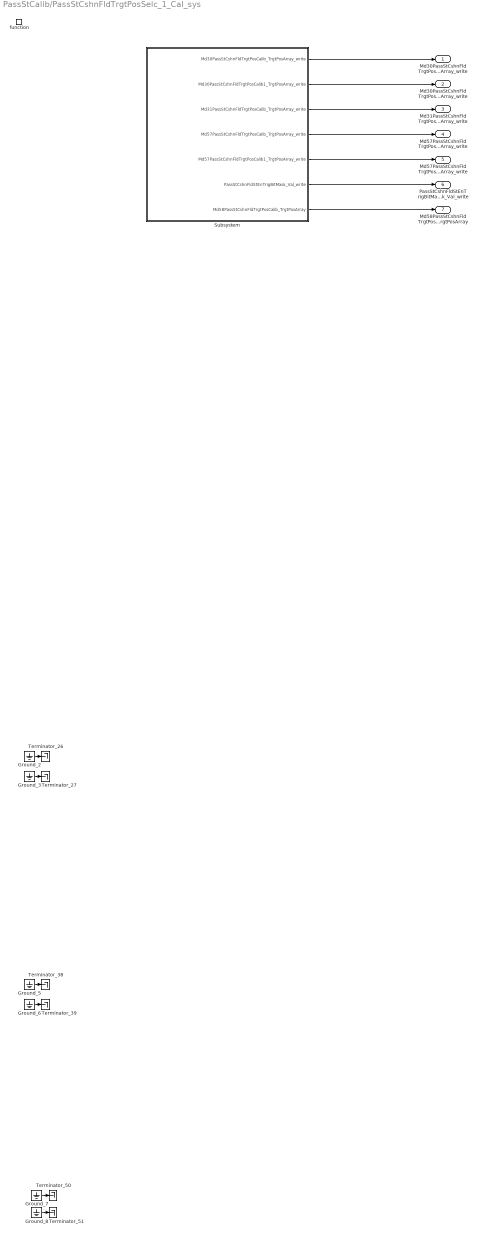
== system PassStCalib/PassStCshnFldTrgtPosSelc_1_Cal_sys ==
  function : TriggerPort  TriggerType=function-call  IsSimulinkFunction=on  FunctionName=PassStCshnFldTrgtPosSelc_1_Cal  VariantControl=(inherit)
  Ground_{2..3,5..8} (6 alike) : Ground
  Subsystem : Subsystem
  Terminator_{26..27,38..39,50..51} (6 alike) : Terminator
  Md30PassStCshnFldTrgtPosCalib_TrgtPosArray_write : Outport  VectorParamsAs1DForOutWhenUnconnected=off
  Md30PassStCshnFldTrgtPosCalib1_TrgtPosArray_write : Outport  Port=2  VectorParamsAs1DForOutWhenUnconnected=off
  Md31PassStCshnFldTrgtPosCalib_TrgtPosArray_write : Outport  Port=3  VectorParamsAs1DForOutWhenUnconnected=off
  Md57PassStCshnFldTrgtPosCalib_TrgtPosArray_write : Outport  Port=4  VectorParamsAs1DForOutWhenUnconnected=off
  Md57PassStCshnFldTrgtPosCalib1_TrgtPosArray_write : Outport  Port=5  VectorParamsAs1DForOutWhenUnconnected=off
  PassStCshnFldStEnTrigBitMask_Val_write : Outport  Port=6  VectorParamsAs1DForOutWhenUnconnected=off
  Md58PassStCshnFldTrgtPosCalib_TrgtPosArray : Outport  Description=|  Port=7  OutDataTypeStr=uint16  PortDimensions=3  VectorParamsAs1DForOutWhenUnconnected=off
      | 0:Pos
      | 1:Max
      | 2:Min
  wires:
  Subsystem/1(Md30PassStCshnFldTrgtPosCalib_TrgtPosArray_write) -> Md30PassStCshnFldTrgtPosCalib_TrgtPosArray_write/1
  Subsystem/2(Md30PassStCshnFldTrgtPosCalib1_TrgtPosArray_write) -> Md30PassStCshnFldTrgtPosCalib1_TrgtPosArray_write/1
  Subsystem/3(Md31PassStCshnFldTrgtPosCalib_TrgtPosArray_write) -> Md31PassStCshnFldTrgtPosCalib_TrgtPosArray_write/1
  Subsystem/4(Md57PassStCshnFldTrgtPosCalib_TrgtPosArray_write) -> Md57PassStCshnFldTrgtPosCalib_TrgtPosArray_write/1
  Subsystem/5(Md57PassStCshnFldTrgtPosCalib1_TrgtPosArray_write) -> Md57PassStCshnFldTrgtPosCalib1_TrgtPosArray_write/1
  Subsystem/6(PassStCshnFldStEnTrigBitMask_Val_write) -> PassStCshnFldStEnTrigBitMask_Val_write/1
  Subsystem/7(Md58PassStCshnFldTrgtPosCalib_TrgtPosArray) -> Md58PassStCshnFldTrgtPosCalib_TrgtPosArray/1
  Ground_2/1 -> Terminator_26/1
  Ground_3/1 -> Terminator_27/1
  Ground_5/1 -> Terminator_38/1
  Ground_6/1 -> Terminator_39/1
  Ground_7/1 -> Terminator_50/1
  Ground_8/1 -> Terminator_51/1
